simulink model "DemoC2D"  (R2014a)
settings: Solver=ode3  StartTime=0.0  StopTime=10.0  FixedStep=0.1  RelTol=1e-3
values from neighbouring files (symbols this model uses):
  G = tf(numK,denK)    [RongKutta.m]
undefined symbols (not defined in the file or in its folder): GD
settings Model: Creator=李广文  LastModifiedBy=李广文

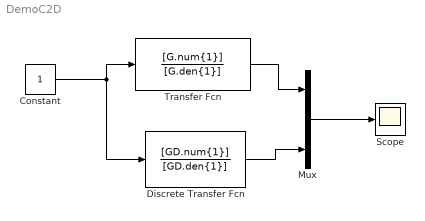
== system DemoC2D ==
  Constant : Constant
  Discrete Transfer Fcn : DiscreteTransferFcn  Numerator=[GD.num{1}]  Denominator=[GD.den{1}]
  Mux : Mux  Inputs=3
  Scope : Scope
  Transfer Fcn : TransferFcn  Numerator=[G.num{1}]  Denominator=[G.den{1}]
  wires:
  Constant/1 -> Discrete Transfer Fcn/1, Transfer Fcn/1
  Mux/1 -> Scope/1
  Transfer Fcn/1 -> Mux/1
  Discrete Transfer Fcn/1 -> Mux/3
